simulink model "DSM_example"  (R2018a)
settings: Solver=VariableStepAuto  StartTime=0.0  StopTime=0.1  RelTol=1e-3
settings Model: Creator=86188  LastModifiedBy=86188

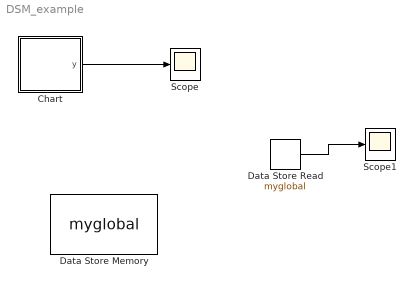
== system DSM_example ==
  Chart : Stateflow chart  TreatAsAtomicUnit=on
  Data Store Memory : DataStoreMemory  DataStoreName=myglobal  ReadBeforeWriteMsg=warning  WriteAfterWriteMsg=warning  WriteAfterReadMsg=warning  InitialValue=[0,0]  ShowAdditionalParam=off  OutDataTypeStr=double
  Data Store Read : DataStoreRead  DataStoreName=myglobal
  Scope : Scope
  Scope1 : Scope
  wires:
  Chart/1(y) -> Scope/1
  Data Store Read/1 -> Scope1/1

== stateflow chart DSM_example/Chart ==
  state A
    en:[myglobal(1)]=duA();
    during:
    myglobal(1) = myglobal(1) +1;
    y=myglobal(1) ;
  state B
    en:myglobal(2)=0;
    during:
    myglobal(2)= myglobal(2)-1;
    y=myglobal(2);
  (default) -> A
  A -> B : [u<0]
  B -> A : [u>=0]
  data: y1 function_output; y output =0; myglobal data_store_memory; u local =2; x local
  function y1 =duA:
    | function y1 =duA
    | y1=3;
